simulink model "Mdl_Tacho"  (R2024b)
settings: Solver=FixedStepDiscrete  StartTime=0.0  StopTime=10.0  FixedStep=0.1  RelTol=1e-3  EnableMultiTasking=on
values from neighbouring files (symbols this model uses):
  EQUIPPED_FLAG = mpt.Parameter    [Mdl_Tacho_DD.m]
  HV_NE = mpt.Parameter    [Mdl_Tacho_DD.m]
  MCUID0025 = mpt.Parameter    [Mdl_Tacho_DD.m]
  MCUID0025_MAX = mpt.Parameter    [Mdl_Tacho_DD.m]
  MCUID0639 = mpt.Parameter    [Mdl_Tacho_DD.m]
  MCUID0640 = mpt.Parameter    [Mdl_Tacho_DD.m]
  Mdl_Tacho_cTaskPeriod = mpt.Parameter    [Mdl_Tacho_rte_types.m]
  N1 = mpt.Parameter    [Mdl_Tacho_DD.m]
  N2 = mpt.Parameter    [Mdl_Tacho_DD.m]
  NE1 = mpt.Parameter    [Mdl_Tacho_DD.m]
  NE_MET = mpt.Parameter    [Mdl_Tacho_DD.m]
  NE_MET_INVALID = mpt.Parameter    [Mdl_Tacho_DD.m]
  PTSYS_48V = mpt.Parameter    [Mdl_Tacho_DD.m]
  PTSYS_CONV = mpt.Parameter    [Mdl_Tacho_DD.m]
  PTSYS_DEFAULT = mpt.Parameter    [Mdl_Tacho_DD.m]
  PTSYS_HV = mpt.Parameter    [Mdl_Tacho_DD.m]
  PTSYS_MOTORHV = mpt.Parameter    [Mdl_Tacho_DD.m]
  PTSYS_PHV = mpt.Parameter    [Mdl_Tacho_DD.m]
  PTSYS_S_S = mpt.Parameter    [Mdl_Tacho_DD.m]
  REDZONE_MAX_VAL = mpt.Parameter    [Mdl_Tacho_DD.m]
  REDZONE_MIN_VAL = mpt.Parameter    [Mdl_Tacho_DD.m]
  RTE_E_MAX_AGE_EXCEEDED = mpt.Parameter    [Mdl_Tacho_rte_types.m]
  RTE_E_NEVER_RECEIVED = mpt.Parameter    [Mdl_Tacho_rte_types.m]
  RTE_E_OK = mpt.Parameter    [Mdl_Tacho_rte_types.m]
  RZ_INIT_VAL = mpt.Parameter    [Mdl_Tacho_DD.m]
  SPD_THRESHOLD = mpt.Parameter    [Mdl_Tacho_DD.m]
  TACHO_070D = mpt.Parameter    [Mdl_Tacho_DD.m]
  TACHO_COUNT_INIT = mpt.Parameter    [Mdl_Tacho_DD.m]
  TACHO_COUNT_INIT_U16 = mpt.Parameter    [Mdl_Tacho_DD.m]
  TACHO_COUNT_ONE = mpt.Parameter    [Mdl_Tacho_DD.m]
  TACHO_COUNT_TWO = mpt.Parameter    [Mdl_Tacho_DD.m]
  TACHO_DEBOUNCE_TIME = mpt.Parameter    [Mdl_Tacho_DD.m]
  TACHO_DISABLE = mpt.Parameter    [Mdl_Tacho_DD.m]
  TACHO_ENABLE = mpt.Parameter    [Mdl_Tacho_DD.m]
  TACHO_F = mpt.Parameter    [Mdl_Tacho_DD.m]
  TACHO_FSPORT = mpt.Parameter    [Mdl_Tacho_DD.m]
  TACHO_GR = mpt.Parameter    [Mdl_Tacho_DD.m]
  TACHO_GRMN = mpt.Parameter    [Mdl_Tacho_DD.m]
  TACHO_HYS_MAX = mpt.Parameter    [Mdl_Tacho_DD.m]
  TACHO_HYS_MIN = mpt.Parameter    [Mdl_Tacho_DD.m]
  TACHO_OFF = mpt.Parameter    [Mdl_Tacho_DD.m]
  TACHO_ON = mpt.Parameter    [Mdl_Tacho_DD.m]
  TACHO_RES_DIVIDER = mpt.Parameter    [Mdl_Tacho_DD.m]
  TACHO_RESOLUTION = mpt.Parameter    [Mdl_Tacho_DD.m]
  TACHO_REV_PEAK_TIMER_ELAPSED = mpt.Parameter    [Mdl_Tacho_DD.m]
  TACHO_RPM_THRESHOLD = mpt.Parameter    [Mdl_Tacho_DD.m]
  TACHO_TEN = mpt.Parameter    [Mdl_Tacho_DD.m]
  TACHO_THRESHOLD = mpt.Parameter    [Mdl_Tacho_DD.m]
  TACHO_VAL_ONE = mpt.Parameter    [Mdl_Tacho_DD.m]
  TACHO_VAL_ONE_U16 = mpt.Parameter    [Mdl_Tacho_DD.m]
  TACHO_VAL_TEN = mpt.Parameter    [Mdl_Tacho_DD.m]
  TACHO_VAL_THREE = mpt.Parameter    [Mdl_Tacho_DD.m]
  TACHO_VAL_TWENTY = mpt.Parameter    [Mdl_Tacho_DD.m]
  TACHO_VAL_ZERO = mpt.Parameter    [Mdl_Tacho_DD.m]
  TACHO_VAL_ZERO_U16 = mpt.Parameter    [Mdl_Tacho_DD.m]
  TACHO_VAL_ZERO_U32 = mpt.Parameter    [Mdl_Tacho_DD.m]
  VAL_ONE = mpt.Parameter    [Mdl_Tacho_DD.m]
  VAL_ZERO = mpt.Parameter    [Mdl_Tacho_DD.m]
undefined symbols (not defined in the file or in its folder): CLUSTER_ACTIVE, CLUSTER_INACTIVE, eEngineSpeedIn, eFUNC_NORTH_AMERICA, eJust_Received, eSIGNAL_MISSING, eSIGNAL_NEVER_RECEIVED, IgnOff, IgnOn, NE1_Recieve_Notify_Value, NE1_SignalVal, pJustRcvdStatus, RxCan_SignalClearJustRcvdStatus, RxCan_SignalGetJustRcvdStatus, RxCan_SignalInvalidProcessingControl, RxCan_SignalMissingProcessingControl, RxCan_SignalNRProcessingControl, SignalId, Status, tRxSignalId_type_instance, tRxSignalJustRcvdStatus_type_instance, tRxSignalStatus_type_instance
libraries: simulink x23
(part 1 of 3)
settings Model: Creator=AELANGO6  LastModifiedBy=AELANGO6
settings DataIOCC: SaveOutput=off
settings OptimizationCC: DefaultParameterBehavior=Inlined  EnhancedBackFolding=on  PassReuseOutputArgsAs=Individual arguments  ZeroExternalMemoryAtStartup=off  ZeroInternalMemoryAtStartup=off  MaxStackSize=750  OptimizeBlockOrder=speed  DifferentSizesBufferReuse=on  OptimizationCustomize=off  EfficientTunableParamExpr=on
settings DebuggingCC: ParameterTunabilityLossMsg=error
settings SFSimCC: MATLABDynamicMemAlloc=off
settings RTWCC: Description=AUTOSAR  SystemTargetFile=autosar.tlc  GenCodeOnly=on  TemplateMakefile=ert_default_tmf  PortableWordSizes=on  DataTypeReplacement=CDataTypesFixedWidth
settings CodeAppCC: ForceParamTrailComments=on  IgnoreCustomStorageClasses=off  OperatorAnnotations=on  SimulinkDataObjDesc=on  SFDataObjDesc=on  InsertBlockDesc=on
settings STFCustomTargetCC: TargetLangStandard=C99 (ISO)  MultiwordLength=256  ParMdlRefBuildCompliant=on  CompOptLevelCompliant=on  IncludeMdlTerminateFcn=off  CombineOutputUpdateFcns=on  SuppressErrorStatus=on  ERTCustomFileBanners=on  SupportNonFinite=off  SupportComplex=off  SupportContinuousTime=off  SupportNonInlinedSFcns=off  RemoveResetFunc=on  ParenthesesLevel=Maximum  CastingMode=Standards  MATLABClassNameForMDSCustomization=Simulink.SoftwareTarget.ERTCustomization  AutosarCompliant=on  UseToolchainInfoCompliant=on  LookupTableObjectStructAxisOrder=2,1,3,4,...  LUTObjectStructOrderEvenSpacing=Size,Table,Breakpoints  SystemTargetFile=autosar.tlc
settings ERTTargetCC: TargetLangStandard=C99 (ISO)  ConcurrentExecutionCompliant=off  IncludeMdlTerminateFcn=off  SuppressErrorStatus=on  SupportNonFinite=off  SupportComplex=off  ParenthesesLevel=Maximum  CastingMode=Standards  ModelStepFunctionPrototypeControlCompliant=off  CPPClassGenCompliant=off  AutosarCompliant=on  LookupTableObjectStructAxisOrder=2,1,3,4,...  LUTObjectStructOrderEvenSpacing=Size,Table,Breakpoints  ERTCustomFileTemplate=example_file_process.tlc  ERTFilePackagingFormat=CompactWithDataFile  BooleanTrueId=TRUE  BooleanFalseId=FALSE

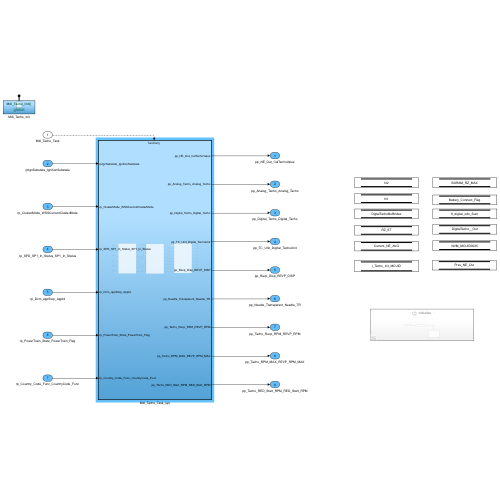
[thumbnail: Simulink's stored preview of the top-level diagram]
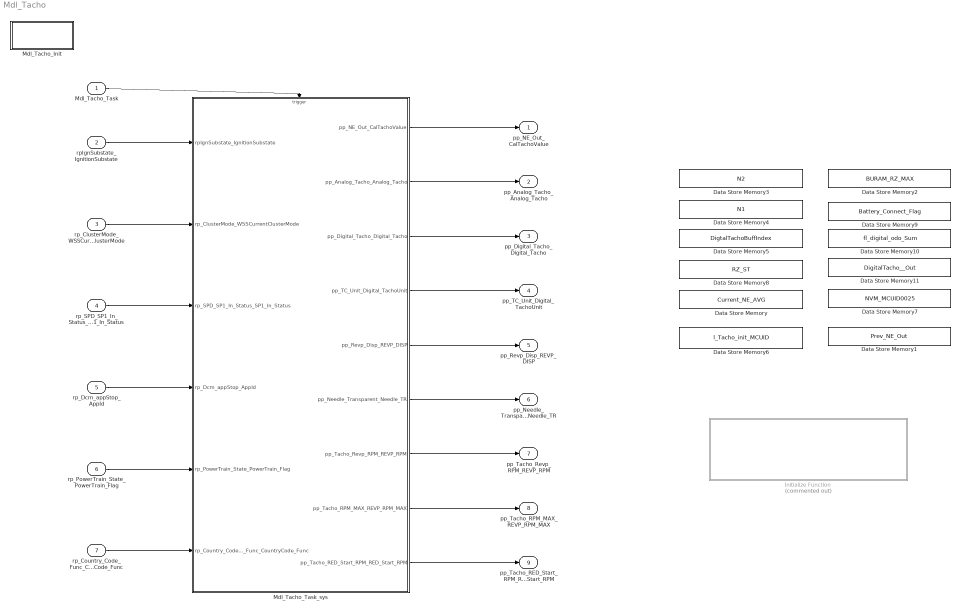
== system Mdl_Tacho ==
  Mdl_Tacho_Task : Inport  SampleTime=0.1  OutputFunctionCall=on
  rpIgnSubstate_IgnitionSubstate : Inport  Port=2  OutDataTypeStr=IgntionSubstateType  PortDimensions=1
  rp_ClusterMode_WSSCurrentClusterMode : Inport  Port=3  OutDataTypeStr=ClusterModes  PortDimensions=1
  rp_SPD_SP1_In_Status_SP1_In_Status : Inport  Port=4  OutDataTypeStr=uint16  PortDimensions=1
  rp_Dcm_appStop_AppId : Inport  Port=5  OutDataTypeStr=IOCtrl_Type  PortDimensions=1
  rp_PowerTrain_State_PowerTrain_Flag : Inport  Port=6  OutDataTypeStr=uint8  PortDimensions=1
  rp_Country_Code_Func_CountryCode_Func : Inport  Port=7  OutDataTypeStr=CountryCode_FuncType  PortDimensions=1
  Data Store Memory : DataStoreMemory  DataStoreName=Current_NE_AVG  ReadBeforeWriteMsg=warning  WriteAfterWriteMsg=warning  WriteAfterReadMsg=warning  InitialValue=NE_AVG_INIT  ShowAdditionalParam=off
  Data Store Memory1 : DataStoreMemory  DataStoreName=Prev_NE_Out  ReadBeforeWriteMsg=warning  WriteAfterWriteMsg=warning  WriteAfterReadMsg=warning  InitialValue=NE_AVG_INIT  ShowAdditionalParam=off
  Data Store Memory10 : DataStoreMemory  DataStoreName=fl_digital_odo_Sum  ReadBeforeWriteMsg=warning  WriteAfterWriteMsg=warning  WriteAfterReadMsg=warning  InitialValue=TACHO_VAL_ZERO_U32  ShowAdditionalParam=off  OutDataTypeStr=uint32
  Data Store Memory11 : DataStoreMemory  DataStoreName=DigitalTacho__Out  ReadBeforeWriteMsg=warning  WriteAfterWriteMsg=warning  WriteAfterReadMsg=warning  InitialValue=TACHO_VAL_ZERO_U16  ShowAdditionalParam=off  OutDataTypeStr=uint16
  Data Store Memory2 : DataStoreMemory  DataStoreName=BURAM_RZ_MAX  ReadBeforeWriteMsg=warning  WriteAfterWriteMsg=warning  WriteAfterReadMsg=warning  ShowAdditionalParam=off
  Data Store Memory3 : DataStoreMemory  DataStoreName=N2  ReadBeforeWriteMsg=warning  WriteAfterWriteMsg=warning  WriteAfterReadMsg=warning  InitialValue=N2  ShowAdditionalParam=off  OutDataTypeStr=uint16
  Data Store Memory4 : DataStoreMemory  DataStoreName=N1  ReadBeforeWriteMsg=warning  WriteAfterWriteMsg=warning  WriteAfterReadMsg=warning  InitialValue=N1  ShowAdditionalParam=off  OutDataTypeStr=uint16
  Data Store Memory5 : DataStoreMemory  DataStoreName=DigtalTachoBuffIndex  ReadBeforeWriteMsg=warning  WriteAfterWriteMsg=warning  WriteAfterReadMsg=warning  InitialValue=TACHO_COUNT_INIT  ShowAdditionalParam=off  OutDataTypeStr=uint8
  Data Store Memory6 : DataStoreMemory  DataStoreName=l_Tacho_init_MCUID  ReadBeforeWriteMsg=warning  WriteAfterWriteMsg=warning  WriteAfterReadMsg=warning  InitialValue=VAL_ZERO  ShowAdditionalParam=off  OutDataTypeStr=uint8
  Data Store Memory7 : DataStoreMemory  DataStoreName=NVM_MCUID0025  ReadBeforeWriteMsg=warning  WriteAfterWriteMsg=warning  WriteAfterReadMsg=warning  InitialValue=TACHO_VAL_ZERO  ShowAdditionalParam=off  OutDataTypeStr=uint8
  Data Store Memory8 : DataStoreMemory  DataStoreName=RZ_ST  ReadBeforeWriteMsg=warning  WriteAfterWriteMsg=warning  WriteAfterReadMsg=warning  InitialValue=RZ_INIT_VAL  ShowAdditionalParam=off  OutDataTypeStr=uint8
  Data Store Memory9 : DataStoreMemory  DataStoreName=Battery_Connect_Flag  ReadBeforeWriteMsg=warning  WriteAfterWriteMsg=warning  WriteAfterReadMsg=warning  ShowAdditionalParam=off  OutDataTypeStr=uint8
  Initialize Function : Subsystem  Commented=on  TreatAsAtomicUnit=on
  Mdl_Tacho_Init : Subsystem  TreatAsAtomicUnit=on
  Mdl_Tacho_Task_sys : Subsystem  TreatAsAtomicUnit=on
  pp_NE_Out_CalTachoValue : Outport  OutDataTypeStr=uint16
  pp_Analog_Tacho_Analog_Tacho : Outport  Port=2  OutDataTypeStr=uint16
  pp_Digital_Tacho_Digital_Tacho : Outport  Port=3  OutDataTypeStr=uint16
  pp_TC_Unit_Digital_TachoUnit : Outport  Port=4  OutDataTypeStr=boolean
  pp_Revp_Disp_REVP_DISP : Outport  Port=5  OutDataTypeStr=boolean
  pp_Needle_Transparent_Needle_TR : Outport  Port=6  OutDataTypeStr=uint8
  pp_Tacho_Revp_RPM_REVP_RPM : Outport  Port=7  OutDataTypeStr=uint16
  pp_Tacho_RPM_MAX_REVP_RPM_MAX : Outport  Port=8  OutDataTypeStr=uint8
  pp_Tacho_RED_Start_RPM_RED_Start_RPM : Outport  Port=9  OutDataTypeStr=uint8
  wires:
  Mdl_Tacho_Task_sys/9(pp_Tacho_RED_Start_RPM_RED_Start_RPM) -> pp_Tacho_RED_Start_RPM_RED_Start_RPM/1
  rp_Country_Code_Func_CountryCode_Func/1 -> Mdl_Tacho_Task_sys/6(rp_Country_Code_Func_CountryCode_Func)
  Mdl_Tacho_Task/1 -> Mdl_Tacho_Task_sys/Trigger
  rp_SPD_SP1_In_Status_SP1_In_Status/1 -> Mdl_Tacho_Task_sys/3(rp_SPD_SP1_In_Status_SP1_In_Status)
  rpIgnSubstate_IgnitionSubstate/1 -> Mdl_Tacho_Task_sys/1(rpIgnSubstate_IgnitionSubstate)
  Mdl_Tacho_Task_sys/3(pp_Digital_Tacho_Digital_Tacho) -> pp_Digital_Tacho_Digital_Tacho/1
  rp_ClusterMode_WSSCurrentClusterMode/1 -> Mdl_Tacho_Task_sys/2(rp_ClusterMode_WSSCurrentClusterMode)
  Mdl_Tacho_Task_sys/6(pp_Needle_Transparent_Needle_TR) -> pp_Needle_Transparent_Needle_TR/1
  rp_Dcm_appStop_AppId/1 -> Mdl_Tacho_Task_sys/4(rp_Dcm_appStop_AppId)
  rp_PowerTrain_State_PowerTrain_Flag/1 -> Mdl_Tacho_Task_sys/5(rp_PowerTrain_State_PowerTrain_Flag)
  Mdl_Tacho_Task_sys/1(pp_NE_Out_CalTachoValue) -> pp_NE_Out_CalTachoValue/1
  Mdl_Tacho_Task_sys/2(pp_Analog_Tacho_Analog_Tacho) -> pp_Analog_Tacho_Analog_Tacho/1
  Mdl_Tacho_Task_sys/4(pp_TC_Unit_Digital_TachoUnit) -> pp_TC_Unit_Digital_TachoUnit/1
  Mdl_Tacho_Task_sys/5(pp_Revp_Disp_REVP_DISP) -> pp_Revp_Disp_REVP_DISP/1
  Mdl_Tacho_Task_sys/7(pp_Tacho_Revp_RPM_REVP_RPM) -> pp_Tacho_Revp_RPM_REVP_RPM/1
  Mdl_Tacho_Task_sys/8(pp_Tacho_RPM_MAX_REVP_RPM_MAX) -> pp_Tacho_RPM_MAX_REVP_RPM_MAX/1

== system Mdl_Tacho/Initialize Function ==
  Compare To Constant3 : simulink/Logic and Bit Operations/Compare To Constant  relop=~=  const=TACHO_VAL_ONE  OutDataTypeStr=boolean
  Data Store Read : DataStoreRead  DataStoreName=Battery_Connect_Flag  IndexOptions=Index vector (dialog)  Indices=1  OutputSizes=1
  Enabled Subsystem : Subsystem  Priority=0  TreatAsAtomicUnit=on
  Event Listener : EventListener  DisableCoverage=on  EventName=reset
  wires:
  Compare To Constant3/1 -> Enabled Subsystem/Enable
  Data Store Read/1 -> Compare To Constant3/1

== system Mdl_Tacho/Mdl_Tacho_Init ==
  Mdl_Tacho_Init : TriggerPort  TriggerType=function-call  IsSimulinkFunction=on  FunctionName=Mdl_Tacho_Init  VariantControl=(inherit)

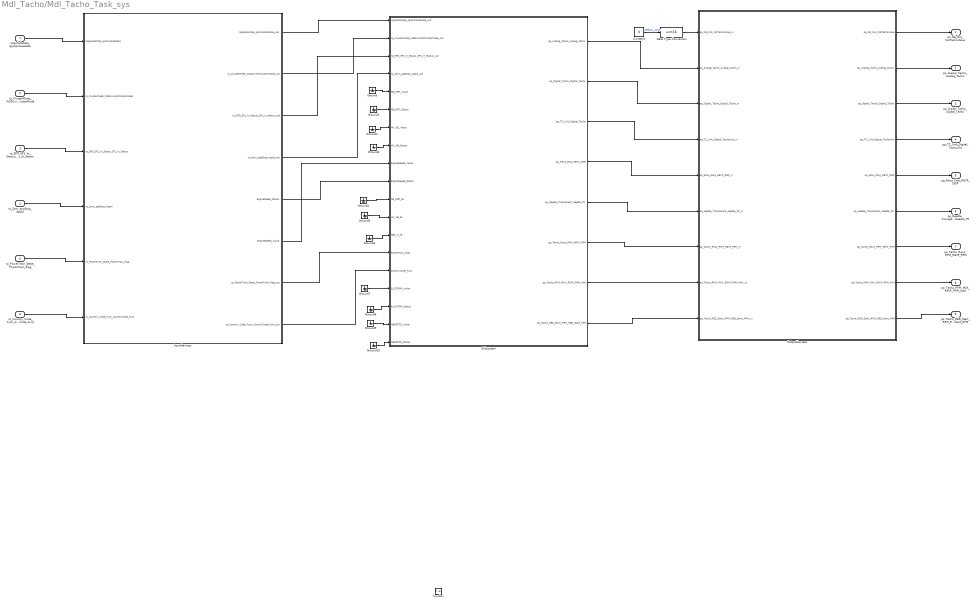
== system Mdl_Tacho/Mdl_Tacho_Task_sys ==
  rpIgnSubstate_IgnitionSubstate : Inport  OutDataTypeStr=IgntionSubstateType  PortDimensions=1
  rp_ClusterMode_WSSCurrentClusterMode : Inport  Port=2  OutDataTypeStr=ClusterModes  PortDimensions=1
  rp_SPD_SP1_In_Status_SP1_In_Status : Inport  Port=3  OutDataTypeStr=uint16  PortDimensions=1
  rp_Dcm_appStop_AppId : Inport  Port=4  OutDataTypeStr=IOCtrl_Type  PortDimensions=1
  rp_PowerTrain_State_PowerTrain_Flag : Inport  Port=5  OutDataTypeStr=uint8  PortDimensions=1
  rp_Country_Code_Func_CountryCode_Func : Inport  Port=6  OutDataTypeStr=CountryCode_FuncType  PortDimensions=1
  function : TriggerPort  TriggerType=function-call  VariantControl=(inherit)  SampleTimeType=periodic  SampleTime=-1
  Constant : Constant  Value=0
  Data Type Conversion : DataTypeConversion  OutDataTypeStr=uint16  SaturateOnIntegerOverflow=off  RndMeth=Floor
  Ground{,1..10} (11 alike) : Ground
  InputHarness : Subsystem  Variant=on
  OutputHarness : Subsystem  Variant=on
  Subsystem : Subsystem
  pp_NE_Out_CalTachoValue : Outport  OutDataTypeStr=uint16  PortDimensions=1
  pp_Analog_Tacho_Analog_Tacho : Outport  Port=2  OutDataTypeStr=uint16  PortDimensions=1
  pp_Digital_Tacho_Digital_Tacho : Outport  Port=3  OutDataTypeStr=uint16  PortDimensions=1
  pp_TC_Unit_Digital_TachoUnit : Outport  Port=4  OutDataTypeStr=boolean  PortDimensions=1
  pp_Revp_Disp_REVP_DISP : Outport  Port=5  OutDataTypeStr=boolean  PortDimensions=1
  pp_Needle_Transparent_Needle_TR : Outport  Port=6  OutDataTypeStr=uint8  PortDimensions=1
  pp_Tacho_Revp_RPM_REVP_RPM : Outport  Port=7  OutDataTypeStr=uint16  PortDimensions=1
  pp_Tacho_RPM_MAX_REVP_RPM_MAX : Outport  Port=8  OutDataTypeStr=uint8  PortDimensions=1
  pp_Tacho_RED_Start_RPM_RED_Start_RPM : Outport  Port=9  OutDataTypeStr=uint8  PortDimensions=1
  wires:
  OutputHarness/1(pp_NE_Out_CalTachoValue) -> pp_NE_Out_CalTachoValue/1
  OutputHarness/2(pp_Analog_Tacho_Analog_Tacho) -> pp_Analog_Tacho_Analog_Tacho/1
  OutputHarness/4(pp_TC_Unit_Digital_TachoUnit) -> pp_TC_Unit_Digital_TachoUnit/1
  rp_ClusterMode_WSSCurrentClusterMode/1 -> InputHarness/2(rp_ClusterMode_WSSCurrentClusterMode)
  OutputHarness/3(pp_Digital_Tacho_Digital_Tacho) -> pp_Digital_Tacho_Digital_Tacho/1
  OutputHarness/5(pp_Revp_Disp_REVP_DISP) -> pp_Revp_Disp_REVP_DISP/1
  OutputHarness/7(pp_Tacho_Revp_RPM_REVP_RPM) -> pp_Tacho_Revp_RPM_REVP_RPM/1
  rp_Dcm_appStop_AppId/1 -> InputHarness/4(rp_Dcm_appStop_AppId)
  OutputHarness/6(pp_Needle_Transparent_Needle_TR) -> pp_Needle_Transparent_Needle_TR/1
  OutputHarness/8(pp_Tacho_RPM_MAX_REVP_RPM_MAX) -> pp_Tacho_RPM_MAX_REVP_RPM_MAX/1
  rp_Country_Code_Func_CountryCode_Func/1 -> InputHarness/6(rp_Country_Code_Func_CountryCode_Func)
  OutputHarness/9(pp_Tacho_RED_Start_RPM_RED_Start_RPM) -> pp_Tacho_RED_Start_RPM_RED_Start_RPM/1
  rpIgnSubstate_IgnitionSubstate/1 -> InputHarness/1(rpIgnSubstate_IgnitionSubstate)
  rp_SPD_SP1_In_Status_SP1_In_Status/1 -> InputHarness/3(rp_SPD_SP1_In_Status_SP1_In_Status)
  rp_PowerTrain_State_PowerTrain_Flag/1 -> InputHarness/5(rp_PowerTrain_State_PowerTrain_Flag)
  InputHarness/1(rpIgnSubstate_IgnitionSubstate_out) -> Subsystem/1(rpIgnSubstate_IgnitionSubstate_out)
  InputHarness/2(rp_ClusterMode_WSSCurrentClusterMode_out) -> Subsystem/2(rp_ClusterMode_WSSCurrentClusterMode_out)
  InputHarness/3(rp_SPD_SP1_In_Status_SP1_In_Status_out) -> Subsystem/3(rp_SPD_SP1_In_Status_SP1_In_Status_out)
  InputHarness/4(rp_Dcm_appStop_AppId_out) -> Subsystem/4(rp_Dcm_appStop_AppId_out)
  InputHarness/7(rp_PowerTrain_State_PowerTrain_Flag_out) -> Subsystem/14(PowerTrain_Flag)
  InputHarness/8(rp_Country_Code_Func_CountryCode_Func_out) -> Subsystem/15(CountryCode_Func)
  Ground3/1 -> Subsystem/8(HV_NE_Status)
  Ground2/1 -> Subsystem/7(HV_NE_Value)
  Ground1/1 -> Subsystem/6(NE_MET_Status)
  Ground/1 -> Subsystem/5(NE_MET_Value)
  Ground4/1 -> Subsystem/11(NE_MET_Ex)
  Ground6/1 -> Subsystem/13(NE1_In_JR)
  Ground5/1 -> Subsystem/12(HV_NE_Ex)
  Ground10/1 -> Subsystem/19(NEMETFD_Status)
  Ground9/1 -> Subsystem/18(NEMETFD_Value)
  Ground8/1 -> Subsystem/17(B_RZRPM_Status)
  Ground7/1 -> Subsystem/16(B_RZRPM_Value)
  Subsystem/2(pp_Digital_Tacho_Digital_Tacho) -> OutputHarness/3(pp_Digital_Tacho_Digital_Tacho_in)
  Subsystem/3(pp_TC_Unit_Digital_Tacho) -> OutputHarness/4(pp_TC_Unit_Digital_TachoUnit_in)
  Subsystem/4(pp_Revp_Disp_REVP_DISP) -> OutputHarness/5(pp_Revp_Disp_REVP_DISP_in)
  Subsystem/5(pp_Needle_Transparent_Needle_TR) -> OutputHarness/6(pp_Needle_Transparent_Needle_TR_in)
  Subsystem/6(pp_Tacho_Revp_RPM_REVP_RPM) -> OutputHarness/7(pp_Tacho_Revp_RPM_REVP_RPM_in)
  Subsystem/7(pp_Tacho_RPM_MAX_REVP_RPM_MAX) -> OutputHarness/8(pp_Tacho_RPM_MAX_REVP_RPM_MAX_in)
  Subsystem/8(pp_Tacho_RED_Start_RPM_RED_Start_RPM) -> OutputHarness/9(pp_Tacho_RED_Start_RPM_RED_Start_RPM_in)
  Subsystem/1(pp_Analog_Tacho_Analog_Tacho) -> OutputHarness/2(pp_Analog_Tacho_Analog_Tacho_in)
  Constant/1 -> Data Type Conversion/1  "Default_value"
  Data Type Conversion/1 -> OutputHarness/1(pp_NE_Out_CalTachoValue_in)
  InputHarness/5(EngineSpeed_Status) -> Subsystem/10(EngineSpeed_Status)
  InputHarness/6(EngineSpeed_Value) -> Subsystem/9(EngineSpeed_Value)

== system Mdl_Tacho/Initialize Function/Enabled Subsystem ==
  Enable : EnablePort
  Constant : Constant  Value=TACHO_VAL_ONE
  Constant10 : Constant  Value=RZ_INIT_VAL
  Data Store Write : DataStoreWrite  DataStoreName=Battery_Connect_Flag  IndexOptions=Index vector (dialog)  Indices=1  OutputSizes=1
  Data Store Write3 : DataStoreWrite  DataStoreName=BURAM_RZ_MAX  IndexOptions=Index vector (dialog)  Indices=1  OutputSizes=1
  wires:
  Constant/1 -> Data Store Write/1
  Constant10/1 -> Data Store Write3/1

== system Mdl_Tacho/Mdl_Tacho_Task_sys/InputHarness ==
  rpIgnSubstate_IgnitionSubstate : Inport  OutDataTypeStr=IgntionSubstateType  PortDimensions=1
  rp_ClusterMode_WSSCurrentClusterMode : Inport  Port=2  OutDataTypeStr=ClusterModes  PortDimensions=1
  rp_SPD_SP1_In_Status_SP1_In_Status : Inport  Port=3  OutDataTypeStr=uint16  PortDimensions=1
  rp_Dcm_appStop_AppId : Inport  Port=4  OutDataTypeStr=IOCtrl_Type  PortDimensions=1
  rp_PowerTrain_State_PowerTrain_Flag : Inport  Port=5  OutDataTypeStr=uint8  PortDimensions=1
  rp_Country_Code_Func_CountryCode_Func : Inport  Port=6  OutDataTypeStr=CountryCode_FuncType  PortDimensions=1
  CodeGeneration : Subsystem  VariantControl=CODEGENERATION
  Simulation : Subsystem  VariantControl=SIMULATION
  rpIgnSubstate_IgnitionSubstate_out : Outport  OutDataTypeStr=IgntionSubstateType  PortDimensions=1
  rp_ClusterMode_WSSCurrentClusterMode_out : Outport  Port=2  OutDataTypeStr=ClusterModes  PortDimensions=1
  rp_SPD_SP1_In_Status_SP1_In_Status_out : Outport  Port=3  OutDataTypeStr=uint16  PortDimensions=1
  rp_Dcm_appStop_AppId_out : Outport  Port=4  OutDataTypeStr=IOCtrl_Type  PortDimensions=1
  EngineSpeed_Status : Outport  Port=5  PortDimensions=1  VectorParamsAs1DForOutWhenUnconnected=off
  EngineSpeed_Value : Outport  Port=6  PortDimensions=1  VectorParamsAs1DForOutWhenUnconnected=off
  rp_PowerTrain_State_PowerTrain_Flag_out : Outport  Port=7  OutDataTypeStr=uint8  PortDimensions=1
  rp_Country_Code_Func_CountryCode_Func_out : Outport  Port=8  OutDataTypeStr=CountryCode_FuncType  PortDimensions=1

== system Mdl_Tacho/Mdl_Tacho_Task_sys/OutputHarness ==
  pp_NE_Out_CalTachoValue_in : Inport  OutDataTypeStr=uint16  PortDimensions=1
  pp_Analog_Tacho_Analog_Tacho_in : Inport  Port=2  OutDataTypeStr=uint16  PortDimensions=1
  pp_Digital_Tacho_Digital_Tacho_in : Inport  Port=3  OutDataTypeStr=uint16  PortDimensions=1
  pp_TC_Unit_Digital_TachoUnit_in : Inport  Port=4  OutDataTypeStr=boolean  PortDimensions=1
  pp_Revp_Disp_REVP_DISP_in : Inport  Port=5  OutDataTypeStr=boolean  PortDimensions=1
  pp_Needle_Transparent_Needle_TR_in : Inport  Port=6  OutDataTypeStr=uint8  PortDimensions=1
  pp_Tacho_Revp_RPM_REVP_RPM_in : Inport  Port=7  OutDataTypeStr=uint16  PortDimensions=1
  pp_Tacho_RPM_MAX_REVP_RPM_MAX_in : Inport  Port=8  OutDataTypeStr=uint8  PortDimensions=1
  pp_Tacho_RED_Start_RPM_RED_Start_RPM_in : Inport  Port=9  OutDataTypeStr=uint8  PortDimensions=1
  CodeGeneration : Subsystem  VariantControl=CODEGENERATION
  Simulation : Subsystem  VariantControl=SIMULATION
  pp_NE_Out_CalTachoValue : Outport  OutDataTypeStr=uint16  PortDimensions=1
  pp_Analog_Tacho_Analog_Tacho : Outport  Port=2  OutDataTypeStr=uint16  PortDimensions=1
  pp_Digital_Tacho_Digital_Tacho : Outport  Port=3  OutDataTypeStr=uint16  PortDimensions=1
  pp_TC_Unit_Digital_TachoUnit : Outport  Port=4  OutDataTypeStr=boolean  PortDimensions=1
  pp_Revp_Disp_REVP_DISP : Outport  Port=5  OutDataTypeStr=boolean  PortDimensions=1
  pp_Needle_Transparent_Needle_TR : Outport  Port=6  OutDataTypeStr=uint8  PortDimensions=1
  pp_Tacho_Revp_RPM_REVP_RPM : Outport  Port=7  OutDataTypeStr=uint16  PortDimensions=1
  pp_Tacho_RPM_MAX_REVP_RPM_MAX : Outport  Port=8  OutDataTypeStr=uint8  PortDimensions=1
  pp_Tacho_RED_Start_RPM_RED_Start_RPM : Outport  Port=9  OutDataTypeStr=uint8  PortDimensions=1

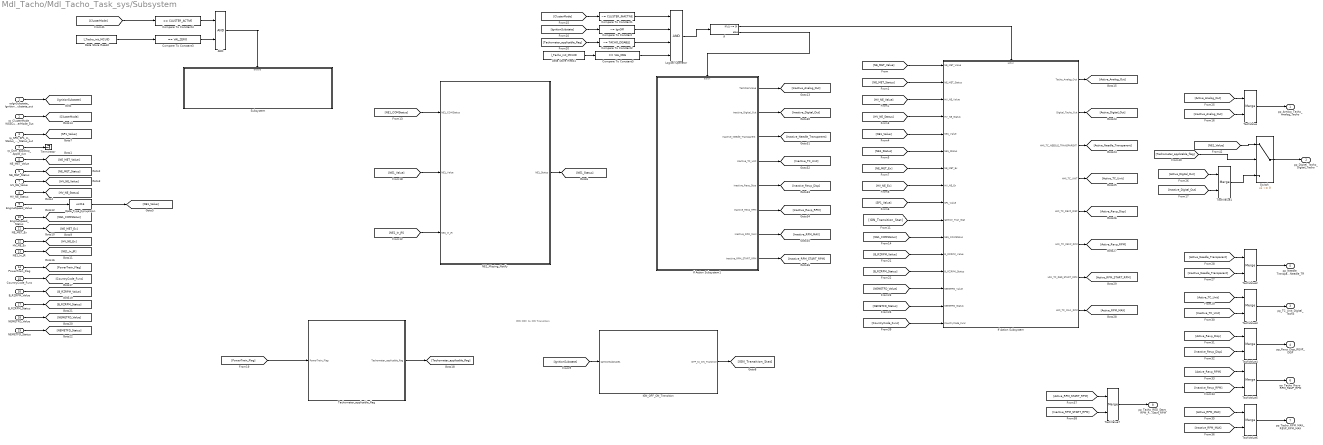
== system Mdl_Tacho/Mdl_Tacho_Task_sys/Subsystem ==
  note: IGN OFF to ON Transition
  rpIgnSubstate_IgnitionSubstate_out : Inport
  rp_ClusterMode_WSSCurrentClusterMode_out : Inport  Port=2
  rp_SPD_SP1_In_Status_SP1_In_Status_out : Inport  Port=3
  rp_Dcm_appStop_AppId_out : Inport  Port=4  OutDataTypeStr=IOCtrl_Type
  NE_MET_Value : Inport  Port=5
  NE_MET_Status : Inport  Port=6
  HV_NE_Value : Inport  Port=7  OutDataTypeStr=uint16
  HV_NE_Status : Inport  Port=8
  EngineSpeed_Value : Inport  Port=9
  EngineSpeed_Status : Inport  Port=10
  NE_MET_Ex : Inport  Port=11
  HV_NE_Ex : Inport  Port=12
  NE1_In_JR : Inport  Port=13
  PowerTrain_Flag : Inport  Port=14
  CountryCode_Func : Inport  Port=15
  B_RZRPM_Value : Inport  Port=16
  B_RZRPM_Status : Inport  Port=17
  NEMETFD_Value : Inport  Port=18
  NEMETFD_Status : Inport  Port=19
  AND : Logic  AllPortsSameDT=off  OutDataTypeStr=boolean
  Compare To Constant : simulink/Logic and Bit Operations/Compare To Constant  relop=~=  const=IgnOff  OutDataTypeStr=boolean
  Compare To Constant1 : simulink/Logic and Bit Operations/Compare To Constant  relop=~=  const=CLUSTER_INACTIVE  OutDataTypeStr=boolean
  Compare To Constant2 : simulink/Logic and Bit Operations/Compare To Constant  relop=~=  const=TACHO_DISABLE  OutDataTypeStr=boolean
  Compare To Constant3 : simulink/Logic and Bit Operations/Compare To Constant  relop===  const=VAL_ZERO  OutDataTypeStr=boolean
  Compare To Constant4 : simulink/Logic and Bit Operations/Compare To Constant  relop===  const=CLUSTER_ACTIVE  OutDataTypeStr=boolean
  Compare To Constant5 : simulink/Logic and Bit Operations/Compare To Constant  relop===  const=VAL_ONE  OutDataTypeStr=boolean
  Data Store Read1 : DataStoreRead  DataStoreName=l_Tacho_init_MCUID  IndexOptions=Index vector (dialog)  Indices=1  OutputSizes=1
  Data Store Read2 : DataStoreRead  DataStoreName=l_Tacho_init_MCUID  IndexOptions=Index vector (dialog)  Indices=1  OutputSizes=1
  Data Type Conversion : DataTypeConversion  OutDataTypeStr=uint16  SaturateOnIntegerOverflow=off  RndMeth=Floor
  IGN_OFF_ON_Transition : Subsystem  TreatAsAtomicUnit=on
      settings: RTWSystemCode=Nonreusable function  RTWFcnNameOpts=Use subsystem name
  If : If  IfExpression=u1 ~= 0
  If Action Subsystem : Subsystem  TreatAsAtomicUnit=on
  If Action Subsystem1 : Subsystem  TreatAsAtomicUnit=on
  Logical Operator : Logic  Inputs=4  AllPortsSameDT=off  OutDataTypeStr=boolean
  NE1_Missing_Notify : Subsystem  TreatAsAtomicUnit=on
      settings: RTWSystemCode=Nonreusable function  RTWFcnNameOpts=Use subsystem name
  Subsystem : Subsystem
  Switch : Switch  Criteria=u2 ~= 0  SaturateOnIntegerOverflow=off  InputSameDT=off
  TachValue{,1..7} (8 alike) : Merge
  Tachometer_applicable_flag : Truth Table  TreatAsAtomicUnit=on
  Terminator : Terminator
  pp_Analog_Tacho_Analog_Tacho : Outport  PortDimensions=1  VectorParamsAs1DForOutWhenUnconnected=off
  pp_Digital_Tacho_Digital_Tacho : Outport  Port=2  PortDimensions=1  VectorParamsAs1DForOutWhenUnconnected=off
  pp_TC_Unit_Digital_Tacho : Outport  Port=3  PortDimensions=1  VectorParamsAs1DForOutWhenUnconnected=off
  pp_Revp_Disp_REVP_DISP : Outport  Port=4  PortDimensions=1  VectorParamsAs1DForOutWhenUnconnected=off
  pp_Needle_Transparent_Needle_TR : Outport  Port=5  PortDimensions=1  VectorParamsAs1DForOutWhenUnconnected=off
  pp_Tacho_Revp_RPM_REVP_RPM : Outport  Port=6  PortDimensions=1  VectorParamsAs1DForOutWhenUnconnected=off
  pp_Tacho_RPM_MAX_REVP_RPM_MAX : Outport  Port=7  PortDimensions=1  VectorParamsAs1DForOutWhenUnconnected=off
  pp_Tacho_RED_Start_RPM_RED_Start_RPM : Outport  Port=8  PortDimensions=1  VectorParamsAs1DForOutWhenUnconnected=off
  wires:
  rpIgnSubstate_IgnitionSubstate_out/1 -> [IgnitionSubstate]
  NE_MET_Value/1 -> [NE_MET_Value]
  NE_MET_Status/1 -> [NE_MET_Status]
  HV_NE_Status/1 -> [HV_NE_Status]
  EngineSpeed_Value/1 -> Data Type Conversion/1
  NE_MET_Ex/1 -> [NE_MET_Ex]
  HV_NE_Ex/1 -> [HV_NE_Ex]
  HV_NE_Value/1 -> [HV_NE_Value]
  [IgnitionSubstate] -> Compare To Constant/1
  If/1 -> If Action Subsystem/Action
  [NE_MET_Value] -> If Action Subsystem/1(NE_MET_Value)
  [NE_MET_Status] -> If Action Subsystem/2(NE_MET_Status)
  [HV_NE_Value] -> If Action Subsystem/3(HV_NE_Value)
  [HV_NE_Status] -> If Action Subsystem/4(HV_NE_Status)
  [NE1_Value] -> If Action Subsystem/5(NE1_Value)
  [NE1_Status] -> If Action Subsystem/6(NE1_Status)
  [NE_MET_Ex] -> If Action Subsystem/7(NE_MET_Ex)
  [HV_NE_Ex] -> If Action Subsystem/8(HV_NE_Ex)
  [SP1_Value] -> If Action Subsystem/9(SP1_Value)
  If/2 -> If Action Subsystem1/Action
  [IgnitionSubstate] -> IGN_OFF_ON_Transition/1(IgnitionSubstate1)
  IGN_OFF_ON_Transition/1(OFF_to_ON_Transtion) -> [IGN_Transition_Stat]
  [IGN_Transition_Stat] -> If Action Subsystem/10(Ignition_Tran_Stat)
  NE1_In_JR/1 -> [NE1_In_JR]
  NE1_Missing_Notify/1(NE1_Status) -> [NE1_Status]
  EngineSpeed_Status/1 -> [NE1_COMStatus]
  [NE1_COMStatus] -> NE1_Missing_Notify/1(NE1_COMStatus)
  [NE1_In_JR] -> NE1_Missing_Notify/3(NE1_In_JR)
  [NE1_COMStatus] -> If Action Subsystem/11(NE1_COMStatus)
  rp_SPD_SP1_In_Status_SP1_In_Status_out/1 -> [SP1_Value]
  rp_ClusterMode_WSSCurrentClusterMode_out/1 -> [ClusterMode]
  [ClusterMode] -> Compare To Constant1/1
  Compare To Constant/1 -> Logical Operator/2
  Logical Operator/1 -> If/1
  If Action Subsystem1/1(TachCalcValue) -> [Inactive_Analog_Out]
  If Action Subsystem/1(Tacho_Analog_Out) -> [Active_Analog_Out]
  [Inactive_Analog_Out] -> TachValue/2
  [Active_Analog_Out] -> TachValue/1
  rp_Dcm_appStop_AppId_out/1 -> Terminator/1
  [NE1_Value] -> NE1_Missing_Notify/2(NE1_Value)
  Compare To Constant1/1 -> Logical Operator/1
  PowerTrain_Flag/1 -> [PowerTrain_Flag]
  CountryCode_Func/1 -> [CountryCode_Func]
  TachValue5/1 -> pp_Tacho_Revp_RPM_REVP_RPM/1
  TachValue3/1 -> pp_TC_Unit_Digital_Tacho/1
  TachValue7/1 -> pp_Tacho_RED_Start_RPM_RED_Start_RPM/1
  TachValue/1 -> pp_Analog_Tacho_Analog_Tacho/1
  TachValue4/1 -> pp_Revp_Disp_REVP_DISP/1
  TachValue6/1 -> pp_Tacho_RPM_MAX_REVP_RPM_MAX/1
  [PowerTrain_Flag] -> Tachometer_applicable_flag/1(PowerTrain_Flag)
  Tachometer_applicable_flag/1(Tachometer_applicable_flag) -> [Tachometer_applicable_flag]
  [Tachometer_applicable_flag] -> Compare To Constant2/1
  Compare To Constant2/1 -> Logical Operator/3
  B_RZRPM_Value/1 -> [B_RZRPM_Value]
  B_RZRPM_Status/1 -> [B_RZRPM_Status]
  NEMETFD_Value/1 -> [NEMETFD_Value]
  NEMETFD_Status/1 -> [NEMETFD_Status]
  [B_RZRPM_Value] -> If Action Subsystem/12(B_RZRPM_Value)
  [B_RZRPM_Status] -> If Action Subsystem/13(B_RZRPM_Status)
  [NEMETFD_Value] -> If Action Subsystem/14(NEMETFD_Value)
  [NEMETFD_Status] -> If Action Subsystem/15(NEMETFD_Status)
  [Active_Digital_Out] -> TachValue1/1
  [Inactive_Digital_Out] -> TachValue1/2
  [Inactive_Needle_Transparent] -> TachValue2/2
  [Active_Needle_Transparent] -> TachValue2/1
  TachValue2/1 -> pp_Needle_Transparent_Needle_TR/1
  [Active_TC_Unit] -> TachValue3/1
  [Inactive_TC_Unit] -> TachValue3/2
  [Active_Revp_Disp] -> TachValue4/1
  [Inactive_Revp_Disp] -> TachValue4/2
  [Active_Revp_RPM] -> TachValue5/1
  [Inactive_Revp_RPM] -> TachValue5/2
  [Active_RPM_MAX] -> TachValue6/1
  [Inactive_RPM_MAX] -> TachValue6/2
  [Active_RPM_START_RPM] -> TachValue7/1
  [Inactive_RPM_START_RPM] -> TachValue7/2
  If Action Subsystem/2(Digital_Tacho_Out) -> [Active_Digital_Out]
  If Action Subsystem/3(HMI_TC_NEEDLE_TRANSPARENT) -> [Active_Needle_Transparent]
  [CountryCode_Func] -> If Action Subsystem/16(CountryCode_Func)
  If Action Subsystem/4(HMI_TC_UNIT) -> [Active_TC_Unit]
  If Action Subsystem/5(HMI_TC_REVP_DISP) -> [Active_Revp_Disp]
  If Action Subsystem/6(HMI_TC_REVP_RPM) -> [Active_Revp_RPM]
  If Action Subsystem/8(HMI_TC_MAX_RPM) -> [Active_RPM_MAX]
  If Action Subsystem/7(HMI_TC_RED_START_RPM) -> [Active_RPM_START_RPM]
  If Action Subsystem1/2(Inactive_Digital_Out) -> [Inactive_Digital_Out]
  If Action Subsystem1/3(Inactive_Needle_Transparent) -> [Inactive_Needle_Transparent]
  If Action Subsystem1/4(Inactive_TC_Unit) -> [Inactive_TC_Unit]
  If Action Subsystem1/5(Inactive_Revp_Disp) -> [Inactive_Revp_Disp]
  If Action Subsystem1/6(Inactive_Revp_RPM) -> [Inactive_Revp_RPM]
  If Action Subsystem1/7(Inactive_RPM_MAX) -> [Inactive_RPM_MAX]
  If Action Subsystem1/8(Inactive_RPM_START_RPM) -> [Inactive_RPM_START_RPM]
  Data Store Read2/1 -> Compare To Constant3/1
  [ClusterMode] -> Compare To Constant4/1
  Compare To Constant3/1 -> AND/2
  AND/1 -> Subsystem/Enable
  Compare To Constant4/1 -> AND/1
  Data Store Read1/1 -> Compare To Constant5/1
  Compare To Constant5/1 -> Logical Operator/4
  Data Type Conversion/1 -> [NE1_Value]
  TachValue1/1 -> Switch/3
  [Tachometer_applicable_flag] -> Switch/2
  [NE1_Value] -> Switch/1
  Switch/1 -> pp_Digital_Tacho_Digital_Tacho/1

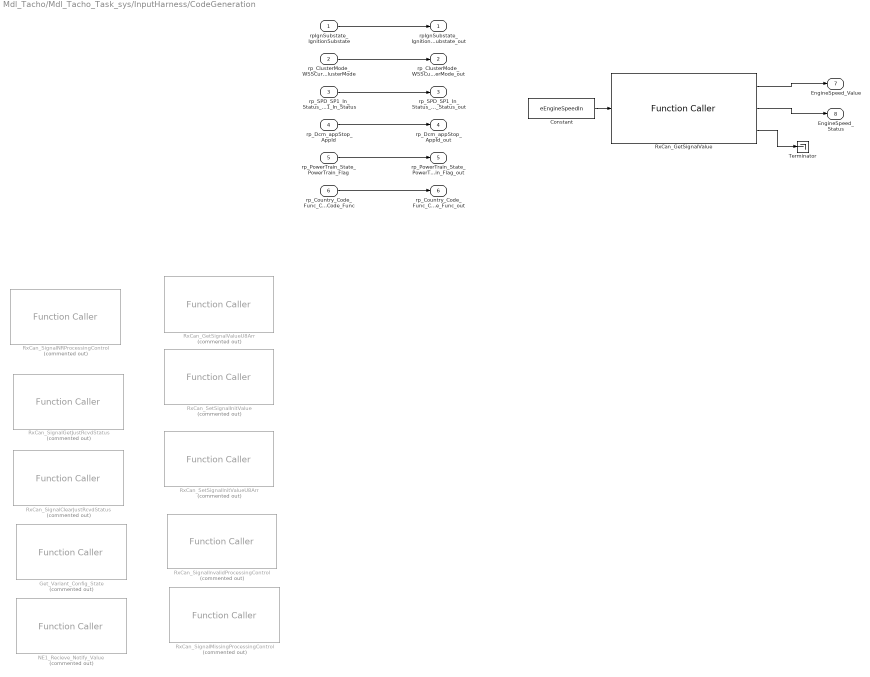
== system Mdl_Tacho/Mdl_Tacho_Task_sys/InputHarness/CodeGeneration ==
  rpIgnSubstate_IgnitionSubstate : Inport  OutDataTypeStr=IgntionSubstateType  PortDimensions=1
  rp_ClusterMode_WSSCurrentClusterMode : Inport  Port=2  OutDataTypeStr=ClusterModes  PortDimensions=1
  rp_SPD_SP1_In_Status_SP1_In_Status : Inport  Port=3  OutDataTypeStr=uint16  PortDimensions=1
  rp_Dcm_appStop_AppId : Inport  Port=4  OutDataTypeStr=IOCtrl_Type  PortDimensions=1
  rp_PowerTrain_State_PowerTrain_Flag : Inport  Port=5  OutDataTypeStr=uint8  PortDimensions=1
  rp_Country_Code_Func_CountryCode_Func : Inport  Port=6  OutDataTypeStr=CountryCode_FuncType  PortDimensions=1
  Constant : Constant  Value=eEngineSpeedIn
  Get_Variant_Config_State : FunctionCaller  Commented=on  FunctionPrototype=VariantActiveSt = Get_Variant_Config_State(VariantID)  InputArgumentSpecifications=uint8(1)  OutputArgumentSpecifications=uint8(1)
  NE1_Recieve_Notify_Value : FunctionCaller  Commented=on  FunctionPrototype=NE1_Recieve_Notify_Value(NE1_SignalVal)  InputArgumentSpecifications=uint16(1)  OutputArgumentSpecifications=<Enter example>
  RxCan_GetSignalValue : FunctionCaller  FunctionPrototype=[pSignalValue,pSignalStatus,error_status] = RxCan_GetSignalValue(SignalId)  InputArgumentSpecifications=tRxSignalId_type_instance(1)  OutputArgumentSpecifications=uint8(1) ,tRxSignalStatus_type_instance(1) ,uint8(1)
  RxCan_GetSignalValueU8Arr : FunctionCaller  Commented=on  FunctionPrototype=[pSignalValue,pSignalStatus,pSignalLength,error_status] = RxCan_GetSignalValueU8Arr(SignalId)  InputArgumentSpecifications=tRxSignalId_type_instance(1)  OutputArgumentSpecifications=uint8(1) ,tRxSignalStatus_type_instance(1) ,uint32(1) ,uint8(1)
  RxCan_SetSignalInitValue : FunctionCaller  Commented=on  FunctionPrototype=[pSignalValue,error_status] = RxCan_SetSignalInitValue(SignalId)  InputArgumentSpecifications=tRxSignalId_type_instance(1)  OutputArgumentSpecifications=uint8(1) ,uint8(1)
  RxCan_SetSignalInitValueU8Arr : FunctionCaller  Commented=on  FunctionPrototype=[pSignaValue,pSignalLength,error_status] = RxCan_SetSignalInitValueU8Arr(SignalId)  InputArgumentSpecifications=tRxSignalId_type_instance(1)  OutputArgumentSpecifications=uint8(1) ,uint32(1) ,uint8(1)
  RxCan_SignalClearJustRcvdStatus : FunctionCaller  Commented=on  FunctionPrototype=RxCan_SignalClearJustRcvdStatus(SignalId)  InputArgumentSpecifications=tRxSignalId_type_instance(1)  OutputArgumentSpecifications=<Enter example>
  RxCan_SignalGetJustRcvdStatus : FunctionCaller  Commented=on  FunctionPrototype=RxCan_SignalGetJustRcvdStatus(SignalId,pJustRcvdStatus)  InputArgumentSpecifications=tRxSignalId_type_instance(1) ,tRxSignalJustRcvdStatus_type_instance(1)  OutputArgumentSpecifications=<Enter example>
  RxCan_SignalInvalidProcessingControl : FunctionCaller  Commented=on  FunctionPrototype=RxCan_SignalInvalidProcessingControl(SignalId,Status)  InputArgumentSpecifications=tRxSignalId_type_instance(1) ,boolean(1)  OutputArgumentSpecifications=<Enter example>
  RxCan_SignalMissingProcessingControl : FunctionCaller  Commented=on  FunctionPrototype=RxCan_SignalMissingProcessingControl(SignalId,Status)  InputArgumentSpecifications=tRxSignalId_type_instance(1) ,boolean(1)  OutputArgumentSpecifications=<Enter example>
  RxCan_SignalNRProcessingControl : FunctionCaller  Commented=on  FunctionPrototype=RxCan_SignalNRProcessingControl(SignalId,Status)  InputArgumentSpecifications=tRxSignalId_type_instance(1) ,boolean(1)  OutputArgumentSpecifications=<Enter example>
  Terminator : Terminator
  rpIgnSubstate_IgnitionSubstate_out : Outport  OutDataTypeStr=IgntionSubstateType  PortDimensions=1
  rp_ClusterMode_WSSCurrentClusterMode_out : Outport  Port=2  OutDataTypeStr=ClusterModes  PortDimensions=1
  rp_SPD_SP1_In_Status_SP1_In_Status_out : Outport  Port=3  OutDataTypeStr=uint16  PortDimensions=1
  rp_Dcm_appStop_AppId_out : Outport  Port=4  OutDataTypeStr=IOCtrl_Type  PortDimensions=1
  rp_PowerTrain_State_PowerTrain_Flag_out : Outport  Port=5  OutDataTypeStr=uint8  PortDimensions=1
  rp_Country_Code_Func_CountryCode_Func_out : Outport  Port=6  OutDataTypeStr=CountryCode_FuncType  PortDimensions=1
  EngineSpeed_Value : Outport  Port=7  PortDimensions=1  VectorParamsAs1DForOutWhenUnconnected=off
  EngineSpeed_Status : Outport  Port=8  PortDimensions=1  VectorParamsAs1DForOutWhenUnconnected=off
  wires:
  rpIgnSubstate_IgnitionSubstate/1 -> rpIgnSubstate_IgnitionSubstate_out/1
  rp_ClusterMode_WSSCurrentClusterMode/1 -> rp_ClusterMode_WSSCurrentClusterMode_out/1
  rp_SPD_SP1_In_Status_SP1_In_Status/1 -> rp_SPD_SP1_In_Status_SP1_In_Status_out/1
  rp_Dcm_appStop_AppId/1 -> rp_Dcm_appStop_AppId_out/1
  rp_PowerTrain_State_PowerTrain_Flag/1 -> rp_PowerTrain_State_PowerTrain_Flag_out/1
  rp_Country_Code_Func_CountryCode_Func/1 -> rp_Country_Code_Func_CountryCode_Func_out/1
  Constant/1 -> RxCan_GetSignalValue/1
  RxCan_GetSignalValue/2 -> EngineSpeed_Status/1
  RxCan_GetSignalValue/1 -> EngineSpeed_Value/1
  RxCan_GetSignalValue/3 -> Terminator/1

== system Mdl_Tacho/Mdl_Tacho_Task_sys/InputHarness/Simulation ==

== system Mdl_Tacho/Mdl_Tacho_Task_sys/OutputHarness/CodeGeneration ==
  pp_NE_Out_CalTachoValue_in : Inport  OutDataTypeStr=uint16  PortDimensions=1
  pp_Analog_Tacho_Analog_Tacho_in : Inport  Port=2  OutDataTypeStr=uint16  PortDimensions=1
  pp_Digital_Tacho_Digital_Tacho_in : Inport  Port=3  OutDataTypeStr=uint16  PortDimensions=1
  pp_TC_Unit_Digital_TachoUnit_in : Inport  Port=4  OutDataTypeStr=boolean  PortDimensions=1
  pp_Revp_Disp_REVP_DISP_in : Inport  Port=5  OutDataTypeStr=boolean  PortDimensions=1
  pp_Needle_Transparent_Needle_TR_in : Inport  Port=6  OutDataTypeStr=uint8  PortDimensions=1
  pp_Tacho_Revp_RPM_REVP_RPM_in : Inport  Port=7  OutDataTypeStr=uint16  PortDimensions=1
  pp_Tacho_RPM_MAX_REVP_RPM_MAX_in : Inport  Port=8  OutDataTypeStr=uint8  PortDimensions=1
  pp_Tacho_RED_Start_RPM_RED_Start_RPM_in : Inport  Port=9  OutDataTypeStr=uint8  PortDimensions=1
  pp_NE_Out_CalTachoValue : Outport  OutDataTypeStr=uint16  PortDimensions=1
  pp_Analog_Tacho_Analog_Tacho : Outport  Port=2  OutDataTypeStr=uint16  PortDimensions=1
  pp_Digital_Tacho_Digital_Tacho : Outport  Port=3  OutDataTypeStr=uint16  PortDimensions=1
  pp_TC_Unit_Digital_TachoUnit : Outport  Port=4  OutDataTypeStr=boolean  PortDimensions=1
  pp_Revp_Disp_REVP_DISP : Outport  Port=5  OutDataTypeStr=boolean  PortDimensions=1
  pp_Needle_Transparent_Needle_TR : Outport  Port=6  OutDataTypeStr=uint8  PortDimensions=1
  pp_Tacho_Revp_RPM_REVP_RPM : Outport  Port=7  OutDataTypeStr=uint16  PortDimensions=1
  pp_Tacho_RPM_MAX_REVP_RPM_MAX : Outport  Port=8  OutDataTypeStr=uint8  PortDimensions=1
  pp_Tacho_RED_Start_RPM_RED_Start_RPM : Outport  Port=9  OutDataTypeStr=uint8  PortDimensions=1
  wires:
  pp_Needle_Transparent_Needle_TR_in/1 -> pp_Needle_Transparent_Needle_TR/1
  pp_Analog_Tacho_Analog_Tacho_in/1 -> pp_Analog_Tacho_Analog_Tacho/1
  pp_Tacho_RPM_MAX_REVP_RPM_MAX_in/1 -> pp_Tacho_RPM_MAX_REVP_RPM_MAX/1
  pp_TC_Unit_Digital_TachoUnit_in/1 -> pp_TC_Unit_Digital_TachoUnit/1
  pp_Tacho_Revp_RPM_REVP_RPM_in/1 -> pp_Tacho_Revp_RPM_REVP_RPM/1
  pp_Digital_Tacho_Digital_Tacho_in/1 -> pp_Digital_Tacho_Digital_Tacho/1
  pp_Revp_Disp_REVP_DISP_in/1 -> pp_Revp_Disp_REVP_DISP/1
  pp_Tacho_RED_Start_RPM_RED_Start_RPM_in/1 -> pp_Tacho_RED_Start_RPM_RED_Start_RPM/1
  pp_NE_Out_CalTachoValue_in/1 -> pp_NE_Out_CalTachoValue/1

== system Mdl_Tacho/Mdl_Tacho_Task_sys/OutputHarness/Simulation ==
  pp_NE_Out_CalTachoValue : Outport  OutDataTypeStr=uint16  PortDimensions=1
  pp_Analog_Tacho_Analog_Tacho : Outport  Port=2  OutDataTypeStr=uint16  PortDimensions=1
  pp_Digital_Tacho_Digital_Tacho : Outport  Port=3  OutDataTypeStr=uint16  PortDimensions=1
  pp_TC_Unit_Digital_TachoUnit : Outport  Port=4  OutDataTypeStr=boolean  PortDimensions=1
  pp_Revp_Disp_REVP_DISP : Outport  Port=5  OutDataTypeStr=boolean  PortDimensions=1
  pp_Needle_Transparent_Needle_TR : Outport  Port=6  OutDataTypeStr=uint8  PortDimensions=1
  pp_Tacho_Revp_RPM_REVP_RPM : Outport  Port=7  OutDataTypeStr=uint16  PortDimensions=1
  pp_Tacho_RPM_MAX_REVP_RPM_MAX : Outport  Port=8  OutDataTypeStr=uint8  PortDimensions=1
  pp_Tacho_RED_Start_RPM_RED_Start_RPM : Outport  Port=9  OutDataTypeStr=uint8  PortDimensions=1

== system Mdl_Tacho/Mdl_Tacho_Task_sys/Subsystem/IGN_OFF_ON_Transition ==
  IgnitionSubstate1 : Inport
  Constant12 : Constant  Value=IgnOff
  Constant8 : Constant  Value=IgnOn
  Logical Operator11 : Logic  AllPortsSameDT=off  OutDataTypeStr=boolean
  Relational Operator7 : RelationalOperator  Operator===  OutDataTypeStr=boolean  InputSameDT=off
  Relational Operator8 : RelationalOperator  Operator===  OutDataTypeStr=boolean  InputSameDT=off
  Unit Delay5 : UnitDelay  SampleTime=-1  StateName=PrevWUSIgnState  HasFrameUpgradeWarning=on
  OFF_to_ON_Transtion : Outport  VectorParamsAs1DForOutWhenUnconnected=off
  wires:
  Constant8/1 -> Relational Operator7/2
  Unit Delay5/1 -> Relational Operator8/1
  Constant12/1 -> Relational Operator8/2
  Relational Operator7/1 -> Logical Operator11/2
  IgnitionSubstate1/1 -> Unit Delay5/1, Relational Operator7/1
  Logical Operator11/1 -> OFF_to_ON_Transtion/1
  Relational Operator8/1 -> Logical Operator11/1

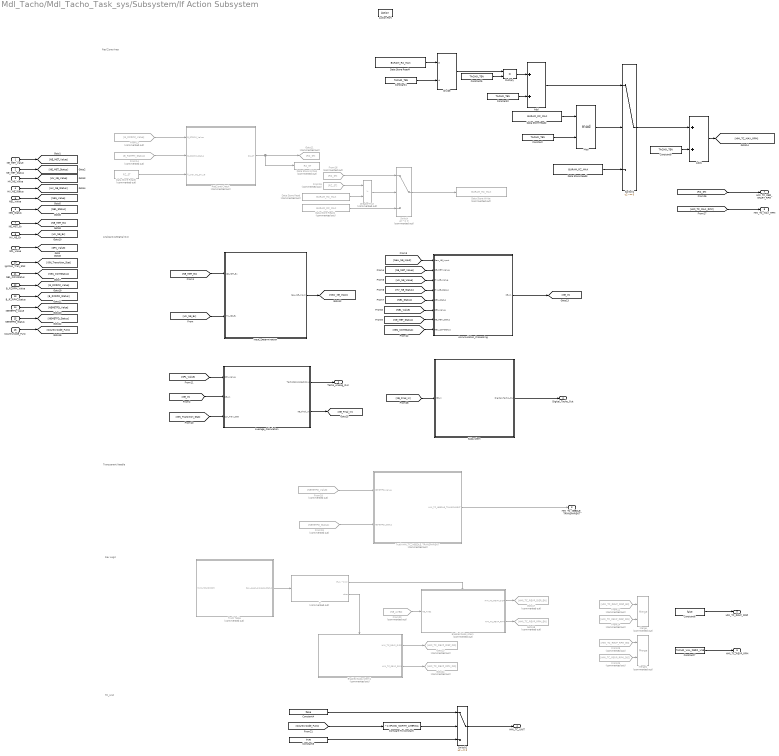
== system Mdl_Tacho/Mdl_Tacho_Task_sys/Subsystem/If Action Subsystem ==
  note: TC_Unit
  note: Rev Logic
  note: Transparent Needle
  note: Red Zone Area
  note: Analog Out/Digital Out
  NE_MET_Value : Inport
  NE_MET_Status : Inport  Port=2
  HV_NE_Value : Inport  Port=3  OutDataTypeStr=uint16
  HV_NE_Status : Inport  Port=4
  NE1_Value : Inport  Port=5
  NE1_Status : Inport  Port=6
  NE_MET_Ex : Inport  Port=7
  HV_NE_Ex : Inport  Port=8
  SP1_Value : Inport  Port=9
  Ignition_Tran_Stat : Inport  Port=10
  NE1_COMStatus : Inport  Port=11
  B_RZRPM_Value : Inport  Port=12
  B_RZRPM_Status : Inport  Port=13
  NEMETFD_Value : Inport  Port=14
  NEMETFD_Status : Inport  Port=15
  CountryCode_Func : Inport  Port=16
  Action Port : ActionPort  ActionPortLabel=if(u1 ~= 0)
  Accumulation_Processing : Subsystem  TreatAsAtomicUnit=on
      settings: RTWSystemCode=Nonreusable function  RTWFcnNameOpts=Use subsystem name
  Add : Sum  AccumDataTypeStr=uint8
  Add1 : Sum  AccumDataTypeStr=uint8
  Average_Calculation : Subsystem  TreatAsAtomicUnit=on  RTWFcnName=Average_Calculation
      settings: RTWSystemCode=Nonreusable function  RTWFcnNameOpts=Use subsystem name
  Compare To Constant : simulink/Logic and Bit Operations/Compare To Constant  relop=~=  const=eFUNC_NORTH_AMERICA  OutDataTypeStr=boolean
  Constant{,1..2,5,8} (5 alike) : Constant  Value=TACHO_TEN
  Constant3 : Constant  Value=true
  Constant4 : Constant  Value=false
  Constant6 : Constant  Value=false
  Constant7 : Constant  Value=TACHO_VAL_ZERO_U16
  Data Store Read : DataStoreRead  Commented=on  DataStoreName=BURAM_RZ_MAX  IndexOptions=Index vector (dialog)  Indices=1  OutputSizes=1
  Data Store Read1 : DataStoreRead  Commented=on  DataStoreName=BURAM_RZ_MAX  IndexOptions=Index vector (dialog)  Indices=1  OutputSizes=1
  Data Store Read2 : DataStoreRead  DataStoreName=BURAM_RZ_MAX  IndexOptions=Index vector (dialog)  Indices=1  OutputSizes=1
  Data Store Read3 : DataStoreRead  DataStoreName=BURAM_RZ_MAX  IndexOptions=Index vector (dialog)  Indices=1  OutputSizes=1
  Data Store Read4 : DataStoreRead  DataStoreName=BURAM_RZ_MAX  IndexOptions=Index vector (dialog)  Indices=1  OutputSizes=1
  Data Store Read6 : DataStoreRead  Commented=on  DataStoreName=RZ_ST  IndexOptions=Index vector (dialog)  Indices=1  OutputSizes=1
  Data Store Write : DataStoreWrite  Commented=on  DataStoreName=BURAM_RZ_MAX  IndexOptions=Index vector (dialog)  Indices=1  OutputSizes=1
  Data Store Write1 : DataStoreWrite  Commented=on  DataStoreName=RZ_ST  IndexOptions=Index vector (dialog)  Indices=1  OutputSizes=1
  Divide : Product  Inputs=*/
  Enabled Subsystem : Subsystem  Commented=on  TreatAsAtomicUnit=on
  Enabled Subsystem1 : Subsystem  Commented=on  TreatAsAtomicUnit=on
  From13 : From  Commented=on  GotoTag=B_RZRPM_Value
  From14 : From  Commented=on  GotoTag=B_RZRPM_Status
  From15 : From  Commented=on  GotoTag=RZ_ST
  From16 : From  Commented=on  GotoTag=RZ_ST
  From18 : From  Commented=on  GotoTag=NEMETFD_Value
  From19 : From  Commented=on  GotoTag=NEMETFD_Status
  From20 : From  Commented=on  GotoTag=NE_AVE2
  From22 : From  Commented=on  GotoTag=HMI_TC_REVP_DISP_EN
  From23 : From  Commented=on  GotoTag=HMI_TC_REVP_RPM_EN
  From24 : From  Commented=on  GotoTag=HMI_TC_REVP_DISP_DIS
  From25 : From  Commented=on  GotoTag=HMI_TC_REVP_RPM_DIS
  Goto11 : Goto  Commented=on  GotoTag=RZ_ST
  Goto17 : Goto  Commented=on  GotoTag=HMI_TC_REVP_DISP_EN
  Goto18 : Goto  Commented=on  GotoTag=HMI_TC_REVP_RPM_EN
  Goto23 : Goto  Commented=on  GotoTag=HMI_TC_REVP_DISP_DIS
  Goto24 : Goto  Commented=on  GotoTag=HMI_TC_REVP_RPM_DIS
  GreaterThan : RelationalOperator  Commented=on  Operator=>  OutDataTypeStr=boolean  RndMeth=Simplest  InputSameDT=off
  If : If  Commented=on  IfExpression=u1 ~= 0
  Input_Determination : Subsystem  TreatAsAtomicUnit=on
      settings: RTWSystemCode=Nonreusable function  RTWFcnNameOpts=Use subsystem name
  Merge : Merge  Commented=on
  Merge1 : Merge  Commented=on
  Mod : Math  Operator=mod  SignedPower=on
  Multiply : Product  OutDataTypeStr=uint8
  RedZone Check : Truth Table  Commented=on  TreatAsAtomicUnit=on
  Subsystem : Subsystem
  Switch : Switch  Commented=on  Criteria=u2 ~= 0  SaturateOnIntegerOverflow=off  InputSameDT=off
  Switch1 : Switch  Criteria=u2 ~= 0  OutDataTypeStr=uint8  SaturateOnIntegerOverflow=off  InputSameDT=off
  Switch2 : Switch  Criteria=u2 ~= 0  SaturateOnIntegerOverflow=off  InputSameDT=off
  Truth HMI_TC_NEEDLE_TRANSPARENT : Truth Table  Commented=on  TreatAsAtomicUnit=on
  Truth Table : Truth Table  Commented=on  TreatAsAtomicUnit=on
  Tacho_Analog_Out : Outport  VectorParamsAs1DForOutWhenUnconnected=off
  Digital_Tacho_Out : Outport  Port=2  VectorParamsAs1DForOutWhenUnconnected=off
  HMI_TC_NEEDLE_TRANSPARENT : Outport  Port=3  VectorParamsAs1DForOutWhenUnconnected=off
  HMI_TC_UNIT : Outport  Port=4  VectorParamsAs1DForOutWhenUnconnected=off
  HMI_TC_REVP_DISP : Outport  Port=5  VectorParamsAs1DForOutWhenUnconnected=off
  HMI_TC_REVP_RPM : Outport  Port=6  VectorParamsAs1DForOutWhenUnconnected=off
  HMI_TC_RED_START_RPM : Outport  Port=7  VectorParamsAs1DForOutWhenUnconnected=off
  HMI_TC_MAX_RPM : Outport  Port=8  VectorParamsAs1DForOutWhenUnconnected=off
  wires:
  [NE_MET_Value] -> Accumulation_Processing/2(NE_MET_Value)
  [HV_NE_Status] -> Accumulation_Processing/4(HV_NE_Status)
  [NE1_Status] -> Accumulation_Processing/5(NE1_Status)
  [HV_NE_Ex] -> Input_Determination/2(HV_NE_Ex)
  [New_NE_Input] -> Accumulation_Processing/1(New_NE_Input)
  Accumulation_Processing/1(NE_In) -> [NE_In]
  [NE_MET_Status] -> Accumulation_Processing/7(NE_MET_Status)
  Input_Determination/1(New_NE_Input) -> [New_NE_Input]
  [NE1_Value] -> Accumulation_Processing/6(NE1_Value)
  [HV_NE_Value] -> Accumulation_Processing/3(HV_NE_Value)
  [NE_MET_Ex] -> Input_Determination/1(NE_MET_Ex)
  NE1_Status/1 -> [NE1_Status]
  HV_NE_Ex/1 -> [HV_NE_Ex]
  NE_MET_Ex/1 -> [NE_MET_Ex]
  HV_NE_Value/1 -> [HV_NE_Value]
  NE1_Value/1 -> [NE1_Value]
  HV_NE_Status/1 -> [HV_NE_Status]
  NE_MET_Value/1 -> [NE_MET_Value]
  NE_MET_Status/1 -> [NE_MET_Status]
  [SP1_Value] -> Average_Calculation/1(SP1_Value)
  [NE_In] -> Average_Calculation/2(NE_In)
  Average_Calculation/1(TachoCalculatedValue) -> Tacho_Analog_Out/1
  SP1_Value/1 -> [SP1_Value]
  Ignition_Tran_Stat/1 -> [IGN_Transition_Stat]
  [IGN_Transition_Stat] -> Average_Calculation/3(Ign_Tran_Stat)
  NE1_COMStatus/1 -> [NE1_COMStatus]
  [NE1_COMStatus] -> Accumulation_Processing/8(NE1_COMStatus)
  B_RZRPM_Value/1 -> [B_RZRPM_Value]
  B_RZRPM_Status/1 -> [B_RZRPM_Status]
  NEMETFD_Value/1 -> [NEMETFD_Value]
  NEMETFD_Status/1 -> [NEMETFD_Status]
  From14/1 -> RedZone Check/2(B_RZRPM_Status)
  RedZone Check/1(RZ_ST) -> Data Store Write1/1, Goto11/1
  From15/1 -> GreaterThan/1
  Data Store Read/1 -> GreaterThan/2
  GreaterThan/1 -> Switch/2
  From16/1 -> Switch/1
  Data Store Read1/1 -> Switch/3
  Switch/1 -> Data Store Write/1
  Constant/1 -> Mod/2
  Data Store Read2/1 -> Mod/1
  Mod/1 -> Switch1/2
  Data Store Read3/1 -> Switch1/3
  Data Store Read4/1 -> Divide/1
  Constant1/1 -> Divide/2
  Constant2/1 -> Add/2
  Add/1 -> Switch1/1
  [NE_Final_In] -> Subsystem/1(NE_In)
  Subsystem/1(Digital_Tacho_Out) -> Digital_Tacho_Out/1
  From19/1 -> Truth HMI_TC_NEEDLE_TRANSPARENT/2(NEMETFD_Status)
  Truth HMI_TC_NEEDLE_TRANSPARENT/1(HMI_TC_NEEDLE_TRANSPARENT) -> HMI_TC_NEEDLE_TRANSPARENT/1
  From20/1 -> Enabled Subsystem/1(NE_AVE2)
  CountryCode_Func/1 -> [CountryCode_Func]
  [CountryCode_Func] -> Compare To Constant/1
  Compare To Constant/1 -> Switch2/2
  Switch2/1 -> HMI_TC_UNIT/1
  Truth Table/1(Rev_peak_process_Status) -> If/1
  If/1 -> Enabled Subsystem/Action
  If/2 -> Enabled Subsystem1/Action
  Enabled Subsystem/1(HMI_TC_REVP_DISP) -> Goto17/1
  Enabled Subsystem/2(HMI_TC_REVP_RPM) -> Goto18/1
  From22/1 -> Merge/1
  From23/1 -> Merge1/1
  Enabled Subsystem1/1(HMI_TC_REVP_DISP) -> Goto23/1
  Enabled Subsystem1/2(HMI_TC_REVP_RPM) -> Goto24/1
  From24/1 -> Merge/2
  From25/1 -> Merge1/2
  [RZ_ST] -> HMI_TC_RED_START_RPM/1
  [HMI_TC_MAX_RPM] -> HMI_TC_MAX_RPM/1
  From18/1 -> Truth HMI_TC_NEEDLE_TRANSPARENT/1(NEMETFD_Value)
  From13/1 -> RedZone Check/1(B_RZRPM_Value)
  Data Store Read6/1 -> RedZone Check/3(fl_prev_RZ_ST_u8)
  Divide/1 -> Multiply/1
  Constant5/1 -> Multiply/2
  Multiply/1 -> Add/1
  Constant3/1 -> Switch2/3
  Constant4/1 -> Switch2/1
  Average_Calculation/2(NE_Final_In) -> [NE_Final_In]
  Constant6/1 -> HMI_TC_REVP_DISP/1
  Constant7/1 -> HMI_TC_REVP_RPM/1
  Constant8/1 -> Add1/2
  Add1/1 -> [HMI_TC_MAX_RPM]
  Switch1/1 -> Add1/1
